simulink model "Simulation_servo_tangage_1_v2_corrige"  (R2013a)
settings: Solver=FixedStepDiscrete  StartTime=0.0  StopTime=inf  RelTol=1e-3
settings Model: Creator=Francois  LastModifiedBy=Propriétaire
settings DataIOCC: SignalLoggingSaveFormat=ModelDataLogs
settings OptimizationCC: ExpressionDepthLimit=2147483647
settings DebuggingCC: FcnCallInpInsideContextMsg=EnableAllAsWarning

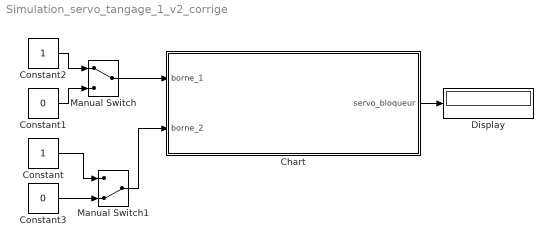
== system Simulation_servo_tangage_1_v2_corrige ==
  Chart : Stateflow chart  TreatAsAtomicUnit=on
  Constant : Constant
  Constant1 : Constant  Value=0
  Constant2 : Constant
  Constant3 : Constant  Value=0
  Display : Display
  Manual Switch : ManualSwitch
  Manual Switch1 : ManualSwitch  CurrentSetting=0
  wires:
  Manual Switch/1 -> Chart/1(borne_1)
  Manual Switch1/1 -> Chart/2(borne_2)
  Constant2/1 -> Manual Switch/1
  Constant1/1 -> Manual Switch/2
  Constant/1 -> Manual Switch1/1
  Constant3/1 -> Manual Switch1/2
  Chart/1(servo_bloqueur) -> Display/1

== stateflow chart Simulation_servo_tangage_1_v2_corrige/Chart ==
  state tangage_bloque
    entry : servo_bloqueur = 45;
  state tangage_libre
    entry : servo_bloqueur = 135;
  state tangage_limite
    entry : servo_bloqueur = 90;
  (default) -> (junction 15)
  (junction 15) -> tangage_libre [order 3] : [borne_1==1 && borne_2==0]
  (junction 15) -> tangage_bloque [order 1] : [borne_1==1 && borne_2==1]
  (junction 15) -> tangage_limite [order 2]
  tangage_libre -> tangage_limite : [borne_1==0 && borne_2==1]
  tangage_bloque -> tangage_limite : [borne_1==0 && borne_2==1]
  tangage_limite -> tangage_libre [order 2] : [borne_1==1 && borne_2==0]
  tangage_limite -> tangage_bloque [order 1] : [borne_1==1 && borne_2==1]
  data: borne_1 input; borne_2 input; servo_bloqueur output double
